simulink model "LTV"  (R2022a)
settings: Solver=VariableStepAuto  StartTime=0.0  StopTime=10.0  RelTol=1e-3
settings Model: Creator=Userx  LastModifiedBy=Userx

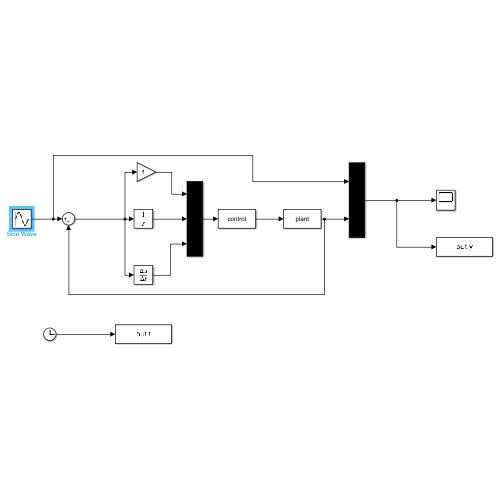
[thumbnail: Simulink's stored preview of the top-level diagram]
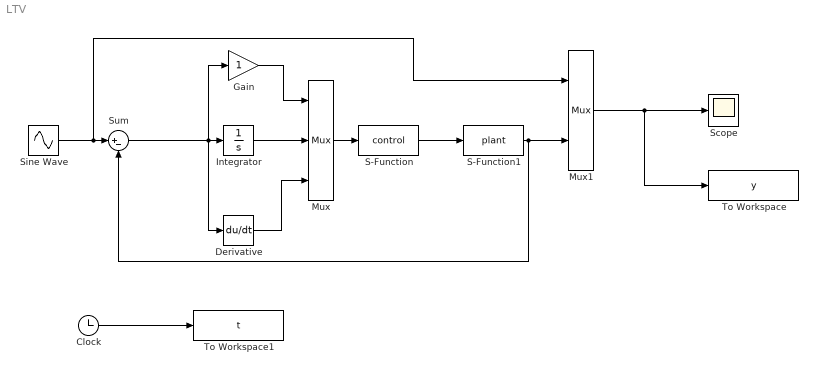
== system LTV ==
  Clock : Clock
  Derivative : Derivative
  Gain : Gain
  Integrator : Integrator
  Mux : Mux  Inputs=3
  Mux1 : Mux  Inputs=2
  S-Function : S-Function  FunctionName=control  SFunctionDeploymentMode=off  EnableBusSupport=off
  S-Function1 : S-Function  FunctionName=plant  SFunctionDeploymentMode=off  EnableBusSupport=off
  Scope : Scope
  Sine Wave : Sin  Amplitude=0.5  Frequency=2*pi  SampleTime=0
  Sum : Sum  Inputs=|+-
  To Workspace : ToWorkspace  VariableName=y  SaveFormat=Timeseries  SampleTime=-1
  To Workspace1 : ToWorkspace  VariableName=t  SaveFormat=Timeseries  SampleTime=-1
  wires:
  Sine Wave/1 -> Mux1/1, Sum/1
  Sum/1 -> Gain/1, Integrator/1, Derivative/1
  Gain/1 -> Mux/1
  Integrator/1 -> Mux/2
  Derivative/1 -> Mux/3
  Mux/1 -> S-Function/1
  S-Function/1 -> S-Function1/1
  S-Function1/1 -> Sum/2, Mux1/2
  Mux1/1 -> Scope/1, To Workspace/1
  Clock/1 -> To Workspace1/1
